simulink model "L5z2"  (R2017a)
settings: Solver=VariableStepAuto  StartTime=0.0  StopTime=16  RelTol=1e-3
settings Model: Creator=DoktorHax  LastModifiedBy=DoktorHax

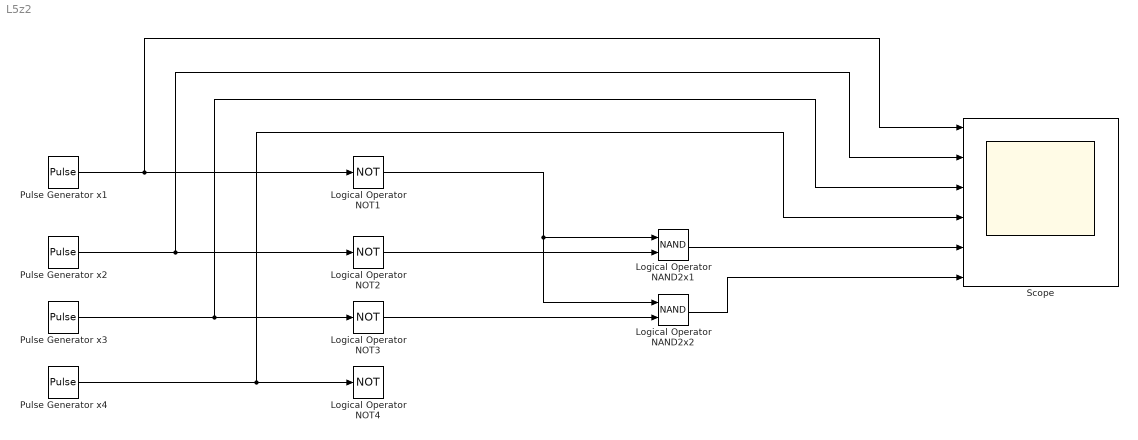
== system L5z2 ==
  Logical Operator NAND2x1 : Logic  Operator=NAND  AllPortsSameDT=off  OutDataTypeStr=boolean
  Logical Operator NAND2x2 : Logic  Operator=NAND  AllPortsSameDT=off  OutDataTypeStr=boolean
  Logical Operator NOT{1..4} (4 alike) : Logic  Operator=NOT  AllPortsSameDT=off  OutDataTypeStr=boolean
  Pulse Generator x1 : DiscretePulseGenerator  PulseType=Time based  PulseWidth=50
  Pulse Generator x2 : DiscretePulseGenerator  PulseType=Time based  Period=4  PulseWidth=50
  Pulse Generator x3 : DiscretePulseGenerator  PulseType=Time based  Period=8  PulseWidth=50
  Pulse Generator x4 : DiscretePulseGenerator  PulseType=Time based  Period=16  PulseWidth=50
  Scope : Scope  NumInputPorts=6
  wires:
  Pulse Generator x2/1 -> Logical Operator NOT2/1, Scope/2
  Logical Operator NOT2/1 -> Logical Operator NAND2x1/2
  Pulse Generator x3/1 -> Logical Operator NOT3/1, Scope/3
  Pulse Generator x4/1 -> Logical Operator NOT4/1, Scope/4
  Pulse Generator x1/1 -> Logical Operator NOT1/1, Scope/1
  Logical Operator NAND2x1/1 -> Scope/5
  Logical Operator NAND2x2/1 -> Scope/6
  Logical Operator NOT1/1 -> Logical Operator NAND2x2/1, Logical Operator NAND2x1/1
  Logical Operator NOT3/1 -> Logical Operator NAND2x2/2
